simulink model "inseguitore_operativo"  (R2024b)
settings: Solver=VariableStepAuto  StartTime=0.0  StopTime=100  RelTol=1e-3
values from neighbouring files (symbols this model uses):
  kd = K(:,3:4)    [regolatore_robot.m]
  kp = K(:,1:2)    [regolatore_robot.m]
  tau = 1    [regolatore_robot.m]
settings Model: Creator=Davide  LastModifiedBy=david
settings OptimizationCC: ReuseModelBlockBuffer=off
settings RTWCC: GPUComputeCapability=3.5

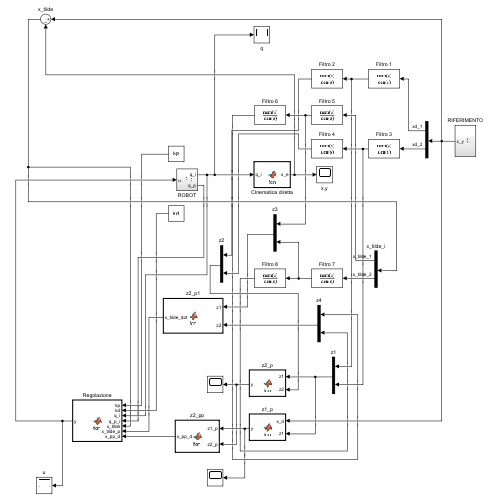
[thumbnail: Simulink's stored preview of the top-level diagram]
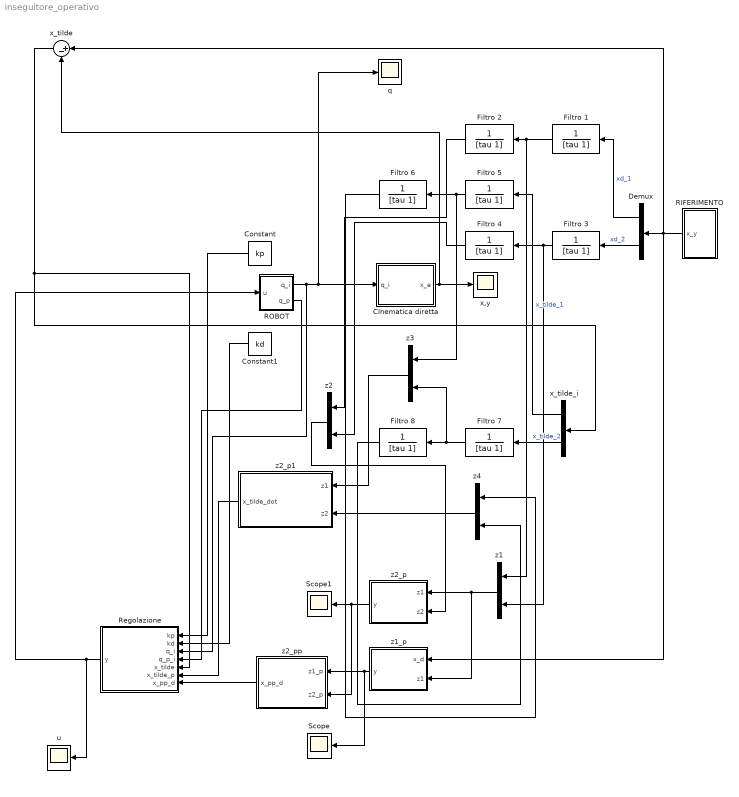
== system inseguitore_operativo ==
  CInematica diretta : MATLAB Function  TreatAsAtomicUnit=on
  Constant : Constant  Value=kp  VectorParams1D=off
  Constant1 : Constant  Value=kd  VectorParams1D=off
  Demux : Demux  Outputs=2
  Filtro {1..8} (8 alike) : TransferFcn  Denominator=[tau 1]
  RIFERIMENTO : Subsystem
  ROBOT : Subsystem
  Regolazione : MATLAB Function  TreatAsAtomicUnit=on
  Scope : Scope
  Scope1 : Scope
  q : Scope
  u : Scope
  x,y : Scope
  x_tilde : Sum  Inputs=|+-
  x_tilde_i : Demux  Outputs=2
  z{1..4} (4 alike) : Mux  Inputs=2
  z1_p : MATLAB Function  TreatAsAtomicUnit=on
  z2_p : MATLAB Function  TreatAsAtomicUnit=on
  z2_p1 : MATLAB Function  TreatAsAtomicUnit=on
  z2_pp : MATLAB Function  TreatAsAtomicUnit=on
  wires:
  x_tilde/1 -> Regolazione/5(x_tilde), x_tilde_i/1
  Regolazione/1(y) -> u/1, ROBOT/1(u)
  Constant/1 -> Regolazione/1(kp)
  Constant1/1 -> Regolazione/2(kd)
  z2_p/1(y) -> z2_pp/2(z2_p), Scope1/1
  ROBOT/1(q_i) -> CInematica diretta/1(q_i), q/1, Regolazione/3(q_i)
  z2_pp/1(x_pp_d) -> Regolazione/7(x_pp_d)
  z2/1 -> z2_p/2(z2)
  z2_p1/1(x_tilde_dot) -> Regolazione/6(x_tilde_p)
  Filtro 6/1 -> z4/1
  ROBOT/2(q_p) -> Regolazione/4(q_p_i)
  z3/1 -> z2_p1/1(z1)
  Filtro 8/1 -> z4/2
  x_tilde_i/2 -> Filtro 7/1  "x_tilde_2"
  z1_p/1(y) -> z2_pp/1(z1_p), Scope/1
  CInematica diretta/1(x_e) -> x_tilde/2, x,y/1
  Filtro 2/1 -> z2/1
  Filtro 5/1 -> Filtro 6/1, z3/1
  Filtro 4/1 -> z2/2
  Filtro 7/1 -> Filtro 8/1, z3/2
  z4/1 -> z2_p1/2(z2)
  z1/1 -> z2_p/1(z1), z1_p/2(z1)
  RIFERIMENTO/1(x_y) -> Demux/1, x_tilde/1, z1_p/1(x_d)
  x_tilde_i/1 -> Filtro 5/1  "x_tilde_1"
  Filtro 1/1 -> Filtro 2/1, z1/1
  Filtro 3/1 -> z1/2, Filtro 4/1
  Demux/2 -> Filtro 3/1  "xd_2"
  Demux/1 -> Filtro 1/1  "xd_1"

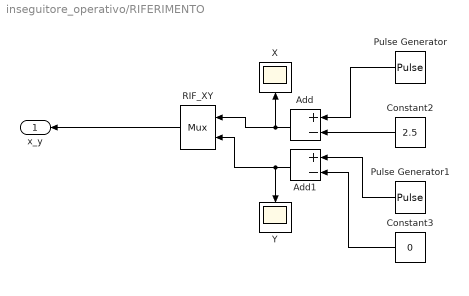
== system inseguitore_operativo/RIFERIMENTO ==
  Add : Sum  Inputs=+-
  Add1 : Sum  Inputs=+-
  Constant2 : Constant  Value=2.5  VectorParams1D=off
  Constant3 : Constant  Value=0  VectorParams1D=off
  Pulse Generator : DiscretePulseGenerator  PulseType=Time based  Amplitude=3.5  Period=10  PulseWidth=50  VectorParams1D=off
  Pulse Generator1 : DiscretePulseGenerator  PulseType=Time based  Period=10  PulseWidth=50  VectorParams1D=off
  RIF_XY : Mux  Inputs=2
      settings: DisplayOption=signals
  X : Scope
  Y : Scope
  x_y : Outport
  wires:
  Add1/1 -> Y/1, RIF_XY/2
  Pulse Generator1/1 -> Add1/1
  Constant3/1 -> Add1/2
  Pulse Generator/1 -> Add/1
  Constant2/1 -> Add/2
  Add/1 -> RIF_XY/1, X/1
  RIF_XY/1 -> x_y/1

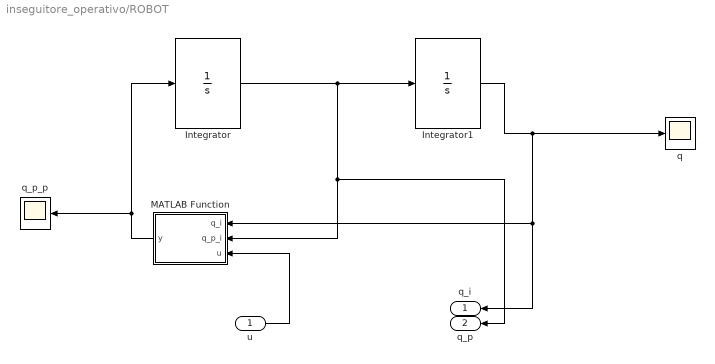
== system inseguitore_operativo/ROBOT ==
  u : Inport
  Integrator : Integrator  InitialCondition=[0;0]
  Integrator1 : Integrator  InitialCondition=[0;0]
  MATLAB Function : MATLAB Function  TreatAsAtomicUnit=on
  q : Scope
  q_p_p : Scope
  q_i : Outport
  q_p : Outport  Port=2
  wires:
  u/1 -> MATLAB Function/3(u)
  Integrator/1 -> q_p/1, MATLAB Function/2(q_p_i), Integrator1/1
  MATLAB Function/1(y) -> Integrator/1, q_p_p/1
  Integrator1/1 -> q_i/1, MATLAB Function/1(q_i), q/1

== matlab function inseguitore_operativo/ROBOT/MATLAB Function ==
  data: q_i input; q_p_i input; u input; y output
function y = fcn(q_i,q_p_i,u)


theta1 = 10.6125; 
theta2 = 0.85; 
theta3 = 2.25;
theta4 = 1.6;
theta5 = 80.9325;
theta6 = 14.7150;
q = q_i;
q_p = q_p_i;
v = u;
F1 = 15;
F2 = 10;

B = [theta1 + 2*theta3*q(2) theta2+theta3*cos(q(2)) ; ...
     theta2+theta3*cos(q(2)) theta4];
C = [-2*theta3*q_p(2)*sin(q(2))  -theta3*q_p(2)*sin(q(2)) ; ...
      theta3*q_p(1)*sin(q(2))              0              ];
g = [theta5*cos(q(1))+theta6*cos(q(1)+q(2)) ; theta6*cos(q(1)+q(2))];
F = [F1*q_p(1) ; F2*q_p(2)];

y = inv(B)*(v - g - F - C*q_p);

== matlab function inseguitore_operativo/Regolazione ==
  data: kp input; kd input; q_i input; q_p_i input; x_tilde input; x_tilde_p input; y output; x_pp_d input
function y = fcn(kp,kd,q_i,q_p_i,x_tilde,x_tilde_p,x_pp_d)

l1=1.5;
l2=1;
q = q_i;
q_p = q_p_i;


%Definizione Jacobiano analitico
J_A = [-l1*sin(q(1))-l2*sin(q(1)+q(2))  -l2*sin(q(1)+q(2));
        l1*cos(q(1))+l2*cos(q(1)+q(2))   l2*cos(q(1)+q(2))];

%Definizione derivata Jacobiano analitico
J_A_dot = [-l1*cos(q(1))*q_p(1)-l2*cos(q(1)+q(2))*(q_p(1)+q_p(2))  -l2*cos(q(1)+q(2))*(q_p(1)+q_p(2));
            l1*sin(q(1))*q_p(1)-l2*sin(q(1)+q(2))*(q_p(1)+q_p(2))  -l2*sin(q(1)+q(2))*(q_p(1)+q_p(2))];


y = inv(J_A)*(x_pp_d+kd*x_tilde_p+kp*x_tilde-J_A_dot*q_p);

== matlab function inseguitore_operativo/z2_p1 ==
  data: z1 input; z2 input; x_tilde_dot output
function x_tilde_dot = fcn(z1,z2)


tau = 1;
z2_p = (-1/tau)*z2+z1;

x_tilde_dot = z2_p;

== matlab function inseguitore_operativo/CInematica diretta ==
  data: q_i input; x_e output
function x_e = fcn(q_i)

q = q_i;
l1 = 1.5;
l2 = 1;

%Estrazione posizione spazio operativo
x_e = [l1*cos(q(1))+l2*cos(q(2)) ; l1*sin(q(1))+l2*sin(q(2))];

== matlab function inseguitore_operativo/z1_p ==
  data: x_d input; z1 input; y output
function y = fcn(x_d,z1)


q = x_d;
tau = 1;
z1_p = (-1/tau)*z1+q;

y = z1_p;

== matlab function inseguitore_operativo/z2_p ==
  data: z1 input; z2 input; y output
function y = fcn(z1,z2)


tau = 1;
z2_p = (-1/tau)*z2+z1;

y = z2_p;

== matlab function inseguitore_operativo/z2_pp ==
  data: z1_p input; z2_p input; x_pp_d output
function x_pp_d = fcn(z1_p,z2_p)



tau = 1;
z2_pp = (-1/tau)*z2_p+z1_p;

x_pp_d = z2_pp;
